simulink model "labFinal_8"  (R2018b)
settings: Solver=FixedStepDiscrete  StartTime=0.0  StopTime=20.0  FixedStep=1  RelTol=1e-3
libraries: hdlsllib x113, simulink_extras x8
(part 4 of 4)

== system labFinal_8/8-Bit_Processor/8-bit Subtractor/2^0/Half_Adder1 ==
  x : Inport
  y : Inport  Port=2
  Calc Carry : Logic  AllPortsSameDT=off  OutDataTypeStr=boolean
  Calc Sum : Logic  Operator=XOR  AllPortsSameDT=off  OutDataTypeStr=boolean
  Sum : Outport
  Carry : Outport  Port=2
  wires:
  Calc Carry/1 -> Carry/1
  x/1 -> Calc Carry/1, Calc Sum/1
  Calc Sum/1 -> Sum/1
  y/1 -> Calc Sum/2, Calc Carry/2

== system labFinal_8/8-Bit_Processor/8-bit Subtractor/2^1/Half_Adder ==
  x : Inport
  y : Inport  Port=2
  Calc Carry : Logic  AllPortsSameDT=off  OutDataTypeStr=boolean
  Calc Sum : Logic  Operator=XOR  AllPortsSameDT=off  OutDataTypeStr=boolean
  Sum : Outport
  Carry : Outport  Port=2
  wires:
  Calc Carry/1 -> Carry/1
  x/1 -> Calc Carry/1, Calc Sum/1
  Calc Sum/1 -> Sum/1
  y/1 -> Calc Sum/2, Calc Carry/2

== system labFinal_8/8-Bit_Processor/8-bit Subtractor/2^1/Half_Adder1 ==
  x : Inport
  y : Inport  Port=2
  Calc Carry : Logic  AllPortsSameDT=off  OutDataTypeStr=boolean
  Calc Sum : Logic  Operator=XOR  AllPortsSameDT=off  OutDataTypeStr=boolean
  Sum : Outport
  Carry : Outport  Port=2
  wires:
  Calc Carry/1 -> Carry/1
  x/1 -> Calc Carry/1, Calc Sum/1
  Calc Sum/1 -> Sum/1
  y/1 -> Calc Sum/2, Calc Carry/2

== system labFinal_8/8-Bit_Processor/8-bit Subtractor/2^2/Half_Adder ==
  x : Inport
  y : Inport  Port=2
  Calc Carry : Logic  AllPortsSameDT=off  OutDataTypeStr=boolean
  Calc Sum : Logic  Operator=XOR  AllPortsSameDT=off  OutDataTypeStr=boolean
  Sum : Outport
  Carry : Outport  Port=2
  wires:
  Calc Carry/1 -> Carry/1
  x/1 -> Calc Carry/1, Calc Sum/1
  Calc Sum/1 -> Sum/1
  y/1 -> Calc Sum/2, Calc Carry/2

== system labFinal_8/8-Bit_Processor/8-bit Subtractor/2^2/Half_Adder1 ==
  x : Inport
  y : Inport  Port=2
  Calc Carry : Logic  AllPortsSameDT=off  OutDataTypeStr=boolean
  Calc Sum : Logic  Operator=XOR  AllPortsSameDT=off  OutDataTypeStr=boolean
  Sum : Outport
  Carry : Outport  Port=2
  wires:
  Calc Carry/1 -> Carry/1
  x/1 -> Calc Carry/1, Calc Sum/1
  Calc Sum/1 -> Sum/1
  y/1 -> Calc Sum/2, Calc Carry/2

== system labFinal_8/8-Bit_Processor/8-bit Subtractor/2^3/Half_Adder ==
  x : Inport
  y : Inport  Port=2
  Calc Carry : Logic  AllPortsSameDT=off  OutDataTypeStr=boolean
  Calc Sum : Logic  Operator=XOR  AllPortsSameDT=off  OutDataTypeStr=boolean
  Sum : Outport
  Carry : Outport  Port=2
  wires:
  Calc Carry/1 -> Carry/1
  x/1 -> Calc Carry/1, Calc Sum/1
  Calc Sum/1 -> Sum/1
  y/1 -> Calc Sum/2, Calc Carry/2

== system labFinal_8/8-Bit_Processor/8-bit Subtractor/2^3/Half_Adder1 ==
  x : Inport
  y : Inport  Port=2
  Calc Carry : Logic  AllPortsSameDT=off  OutDataTypeStr=boolean
  Calc Sum : Logic  Operator=XOR  AllPortsSameDT=off  OutDataTypeStr=boolean
  Sum : Outport
  Carry : Outport  Port=2
  wires:
  Calc Carry/1 -> Carry/1
  x/1 -> Calc Carry/1, Calc Sum/1
  Calc Sum/1 -> Sum/1
  y/1 -> Calc Sum/2, Calc Carry/2

== system labFinal_8/8-Bit_Processor/8-bit Subtractor/2^4/Half_Adder ==
  x : Inport
  y : Inport  Port=2
  Calc Carry : Logic  AllPortsSameDT=off  OutDataTypeStr=boolean
  Calc Sum : Logic  Operator=XOR  AllPortsSameDT=off  OutDataTypeStr=boolean
  Sum : Outport
  Carry : Outport  Port=2
  wires:
  Calc Carry/1 -> Carry/1
  x/1 -> Calc Carry/1, Calc Sum/1
  Calc Sum/1 -> Sum/1
  y/1 -> Calc Sum/2, Calc Carry/2

== system labFinal_8/8-Bit_Processor/8-bit Subtractor/2^4/Half_Adder1 ==
  x : Inport
  y : Inport  Port=2
  Calc Carry : Logic  AllPortsSameDT=off  OutDataTypeStr=boolean
  Calc Sum : Logic  Operator=XOR  AllPortsSameDT=off  OutDataTypeStr=boolean
  Sum : Outport
  Carry : Outport  Port=2
  wires:
  Calc Carry/1 -> Carry/1
  x/1 -> Calc Carry/1, Calc Sum/1
  Calc Sum/1 -> Sum/1
  y/1 -> Calc Sum/2, Calc Carry/2

== system labFinal_8/8-Bit_Processor/8-bit Subtractor/2^5/Half_Adder ==
  x : Inport
  y : Inport  Port=2
  Calc Carry : Logic  AllPortsSameDT=off  OutDataTypeStr=boolean
  Calc Sum : Logic  Operator=XOR  AllPortsSameDT=off  OutDataTypeStr=boolean
  Sum : Outport
  Carry : Outport  Port=2
  wires:
  Calc Carry/1 -> Carry/1
  x/1 -> Calc Carry/1, Calc Sum/1
  Calc Sum/1 -> Sum/1
  y/1 -> Calc Sum/2, Calc Carry/2

== system labFinal_8/8-Bit_Processor/8-bit Subtractor/2^5/Half_Adder1 ==
  x : Inport
  y : Inport  Port=2
  Calc Carry : Logic  AllPortsSameDT=off  OutDataTypeStr=boolean
  Calc Sum : Logic  Operator=XOR  AllPortsSameDT=off  OutDataTypeStr=boolean
  Sum : Outport
  Carry : Outport  Port=2
  wires:
  Calc Carry/1 -> Carry/1
  x/1 -> Calc Carry/1, Calc Sum/1
  Calc Sum/1 -> Sum/1
  y/1 -> Calc Sum/2, Calc Carry/2

== system labFinal_8/8-Bit_Processor/8-bit Subtractor/2^6/Half_Adder ==
  x : Inport
  y : Inport  Port=2
  Calc Carry : Logic  AllPortsSameDT=off  OutDataTypeStr=boolean
  Calc Sum : Logic  Operator=XOR  AllPortsSameDT=off  OutDataTypeStr=boolean
  Sum : Outport
  Carry : Outport  Port=2
  wires:
  Calc Carry/1 -> Carry/1
  x/1 -> Calc Carry/1, Calc Sum/1
  Calc Sum/1 -> Sum/1
  y/1 -> Calc Sum/2, Calc Carry/2

== system labFinal_8/8-Bit_Processor/8-bit Subtractor/2^6/Half_Adder1 ==
  x : Inport
  y : Inport  Port=2
  Calc Carry : Logic  AllPortsSameDT=off  OutDataTypeStr=boolean
  Calc Sum : Logic  Operator=XOR  AllPortsSameDT=off  OutDataTypeStr=boolean
  Sum : Outport
  Carry : Outport  Port=2
  wires:
  Calc Carry/1 -> Carry/1
  x/1 -> Calc Carry/1, Calc Sum/1
  Calc Sum/1 -> Sum/1
  y/1 -> Calc Sum/2, Calc Carry/2

== system labFinal_8/8-Bit_Processor/8-bit Subtractor/2^7/Half_Adder ==
  x : Inport
  y : Inport  Port=2
  Calc Carry : Logic  AllPortsSameDT=off  OutDataTypeStr=boolean
  Calc Sum : Logic  Operator=XOR  AllPortsSameDT=off  OutDataTypeStr=boolean
  Sum : Outport
  Carry : Outport  Port=2
  wires:
  Calc Carry/1 -> Carry/1
  x/1 -> Calc Carry/1, Calc Sum/1
  Calc Sum/1 -> Sum/1
  y/1 -> Calc Sum/2, Calc Carry/2

== system labFinal_8/8-Bit_Processor/8-bit Subtractor/2^7/Half_Adder1 ==
  x : Inport
  y : Inport  Port=2
  Calc Carry : Logic  AllPortsSameDT=off  OutDataTypeStr=boolean
  Calc Sum : Logic  Operator=XOR  AllPortsSameDT=off  OutDataTypeStr=boolean
  Sum : Outport
  Carry : Outport  Port=2
  wires:
  Calc Carry/1 -> Carry/1
  x/1 -> Calc Carry/1, Calc Sum/1
  Calc Sum/1 -> Sum/1
  y/1 -> Calc Sum/2, Calc Carry/2
